simulink model "dual500MHzPFB"  (Simulink 6.2)
settings: Solver=ode45  StartTime=0.0  StopTime=10000  RelTol=1e-3
libraries: xbsIndex_r3 x2070, casper_library x180, xps_library x12, gtkWave x5, gavrt_library x1
(part 16 of 20)

== system dual500MHzPFB/cfgspec/FFT_Subsystem/fft_wideband_real1/fft_unscrambler/square_transposer/barrel_switcher ==
  sel : Inport  Port=1  LatchInput=off
  sync_in : Inport  Port=2  LatchInput=off
  In1 : Inport  Port=3  LatchInput=off
  In2 : Inport  Port=4  LatchInput=off
  Delay_sync : xbsIndex_r3/Delay  latency=1  reg_retiming=off  explicit_period=off  period=1  en=off  accept_only_valid=off  init_zero=on  dbl_ovrd=off  show_param=off
      settings: xl_area=[0, 0, 0, 0, 0, 0, 0]
  Mux11 : xbsIndex_r3/Mux  inputs=2  precision=Full  arith_type="Signed  (2's comp)"  n_bits=8  bin_pt=2  quantization=Truncate  overflow=Wrap  latency=1  explicit_period=off  period=1  en=off  dbl_ovrd=off  show_param=off  mux_type=off  use_rpm=off  gen_core=off
      settings: xl_area=[0, 0, 0, 0, 0, 0, 0]
  Mux21 : xbsIndex_r3/Mux  inputs=2  precision=Full  arith_type="Signed  (2's comp)"  n_bits=8  bin_pt=2  quantization=Truncate  overflow=Wrap  latency=1  explicit_period=off  period=1  en=off  dbl_ovrd=off  show_param=off  mux_type=off  use_rpm=off  gen_core=off
      settings: xl_area=[0, 0, 0, 0, 0, 0, 0]
  Slice1 : xbsIndex_r3/Slice  mode=Upper Bit Location + Width  nbits=1  bit1=-0  base1=MSB of Input  bit0=0  base0=LSB of Input  boolean_output=off  explicit_period=off  period=1  dbl_ovrd=off
  sync_out : Outport
  Out1 : Outport  Port=2
  Out2 : Outport  Port=3
  wires:
  Mux21/1 -> Out2/1
  In2/1 -> Mux11/3, Mux21/2
  Mux11/1 -> Out1/1
  In1/1 -> Mux21/3, Mux11/2
  Slice1/1 -> Mux21/1, Mux11/1
  sel/1 -> Slice1/1
  Delay_sync/1 -> sync_out/1
  sync_in/1 -> Delay_sync/1

== system dual500MHzPFB/cfgspec/PFB_Subsystem/pfb_fir_real/pol1_in1_last_tap/pfb_real_add_tree/adder_tree1 ==
  sync : Inport  Port=1  LatchInput=off
  din1 : Inport  Port=2  LatchInput=off
  din2 : Inport  Port=3  LatchInput=off
  addr1 : xbsIndex_r3/AddSub  mode=Addition  precision=Full  arith_type=Unsigned  n_bits=8  bin_pt=2  quantization=Truncate  overflow=Wrap  latency=2  explicit_period=off  period=1  use_carryin=off  use_carryout=off  en=off  dbl_ovrd=off  show_param=off  use_core=on  pipeline=on  use_rpm=on  gen_core=off
      settings: xl_area=[0, 0, 0, 0, 0, 0, 0]
  sync_delay : xbsIndex_r3/Delay  latency=2  reg_retiming=off  explicit_period=off  period=1  en=off  accept_only_valid=off  init_zero=on  dbl_ovrd=off  show_param=off
      settings: xl_area=[0, 0, 0, 0, 0, 0, 0]
  sync_out : Outport
  dout : Outport  Port=2
  wires:
  sync/1 -> sync_delay/1
  sync_delay/1 -> sync_out/1
  din1/1 -> addr1/1
  din2/1 -> addr1/2
  addr1/1 -> dout/1

== system dual500MHzPFB/cfgspec/PFB_Subsystem/pfb_fir_real/pol1_in2_last_tap/pfb_real_add_tree/adder_tree1 ==
  sync : Inport  Port=1  LatchInput=off
  din1 : Inport  Port=2  LatchInput=off
  din2 : Inport  Port=3  LatchInput=off
  addr1 : xbsIndex_r3/AddSub  mode=Addition  precision=Full  arith_type=Unsigned  n_bits=8  bin_pt=2  quantization=Truncate  overflow=Wrap  latency=2  explicit_period=off  period=1  use_carryin=off  use_carryout=off  en=off  dbl_ovrd=off  show_param=off  use_core=on  pipeline=on  use_rpm=on  gen_core=off
      settings: xl_area=[0, 0, 0, 0, 0, 0, 0]
  sync_delay : xbsIndex_r3/Delay  latency=2  reg_retiming=off  explicit_period=off  period=1  en=off  accept_only_valid=off  init_zero=on  dbl_ovrd=off  show_param=off
      settings: xl_area=[0, 0, 0, 0, 0, 0, 0]
  sync_out : Outport
  dout : Outport  Port=2
  wires:
  sync/1 -> sync_delay/1
  sync_delay/1 -> sync_out/1
  din1/1 -> addr1/1
  din2/1 -> addr1/2
  addr1/1 -> dout/1

== system dual500MHzPFB/cfgspec/PFB_Subsystem/pfb_fir_real/pol1_in3_last_tap/pfb_real_add_tree/adder_tree1 ==
  sync : Inport  Port=1  LatchInput=off
  din1 : Inport  Port=2  LatchInput=off
  din2 : Inport  Port=3  LatchInput=off
  addr1 : xbsIndex_r3/AddSub  mode=Addition  precision=Full  arith_type=Unsigned  n_bits=8  bin_pt=2  quantization=Truncate  overflow=Wrap  latency=2  explicit_period=off  period=1  use_carryin=off  use_carryout=off  en=off  dbl_ovrd=off  show_param=off  use_core=on  pipeline=on  use_rpm=on  gen_core=off
      settings: xl_area=[0, 0, 0, 0, 0, 0, 0]
  sync_delay : xbsIndex_r3/Delay  latency=2  reg_retiming=off  explicit_period=off  period=1  en=off  accept_only_valid=off  init_zero=on  dbl_ovrd=off  show_param=off
      settings: xl_area=[0, 0, 0, 0, 0, 0, 0]
  sync_out : Outport
  dout : Outport  Port=2
  wires:
  sync/1 -> sync_delay/1
  sync_delay/1 -> sync_out/1
  din1/1 -> addr1/1
  din2/1 -> addr1/2
  addr1/1 -> dout/1

== system dual500MHzPFB/cfgspec/PFB_Subsystem/pfb_fir_real/pol1_in4_last_tap/pfb_real_add_tree/adder_tree1 ==
  sync : Inport  Port=1  LatchInput=off
  din1 : Inport  Port=2  LatchInput=off
  din2 : Inport  Port=3  LatchInput=off
  addr1 : xbsIndex_r3/AddSub  mode=Addition  precision=Full  arith_type=Unsigned  n_bits=8  bin_pt=2  quantization=Truncate  overflow=Wrap  latency=2  explicit_period=off  period=1  use_carryin=off  use_carryout=off  en=off  dbl_ovrd=off  show_param=off  use_core=on  pipeline=on  use_rpm=on  gen_core=off
      settings: xl_area=[0, 0, 0, 0, 0, 0, 0]
  sync_delay : xbsIndex_r3/Delay  latency=2  reg_retiming=off  explicit_period=off  period=1  en=off  accept_only_valid=off  init_zero=on  dbl_ovrd=off  show_param=off
      settings: xl_area=[0, 0, 0, 0, 0, 0, 0]
  sync_out : Outport
  dout : Outport  Port=2
  wires:
  sync/1 -> sync_delay/1
  sync_delay/1 -> sync_out/1
  din1/1 -> addr1/1
  din2/1 -> addr1/2
  addr1/1 -> dout/1

== system dual500MHzPFB/cfgspec/PFB_Subsystem/pfb_fir_real1/pol1_in1_last_tap/pfb_real_add_tree/adder_tree1 ==
  sync : Inport  Port=1  LatchInput=off
  din1 : Inport  Port=2  LatchInput=off
  din2 : Inport  Port=3  LatchInput=off
  addr1 : xbsIndex_r3/AddSub  mode=Addition  precision=Full  arith_type=Unsigned  n_bits=8  bin_pt=2  quantization=Truncate  overflow=Wrap  latency=2  explicit_period=off  period=1  use_carryin=off  use_carryout=off  en=off  dbl_ovrd=off  show_param=off  use_core=on  pipeline=on  use_rpm=on  gen_core=off
      settings: xl_area=[0, 0, 0, 0, 0, 0, 0]
  sync_delay : xbsIndex_r3/Delay  latency=2  reg_retiming=off  explicit_period=off  period=1  en=off  accept_only_valid=off  init_zero=on  dbl_ovrd=off  show_param=off
      settings: xl_area=[0, 0, 0, 0, 0, 0, 0]
  sync_out : Outport
  dout : Outport  Port=2
  wires:
  sync/1 -> sync_delay/1
  sync_delay/1 -> sync_out/1
  din1/1 -> addr1/1
  din2/1 -> addr1/2
  addr1/1 -> dout/1

== system dual500MHzPFB/cfgspec/PFB_Subsystem/pfb_fir_real1/pol1_in2_last_tap/pfb_real_add_tree/adder_tree1 ==
  sync : Inport  Port=1  LatchInput=off
  din1 : Inport  Port=2  LatchInput=off
  din2 : Inport  Port=3  LatchInput=off
  addr1 : xbsIndex_r3/AddSub  mode=Addition  precision=Full  arith_type=Unsigned  n_bits=8  bin_pt=2  quantization=Truncate  overflow=Wrap  latency=2  explicit_period=off  period=1  use_carryin=off  use_carryout=off  en=off  dbl_ovrd=off  show_param=off  use_core=on  pipeline=on  use_rpm=on  gen_core=off
      settings: xl_area=[0, 0, 0, 0, 0, 0, 0]
  sync_delay : xbsIndex_r3/Delay  latency=2  reg_retiming=off  explicit_period=off  period=1  en=off  accept_only_valid=off  init_zero=on  dbl_ovrd=off  show_param=off
      settings: xl_area=[0, 0, 0, 0, 0, 0, 0]
  sync_out : Outport
  dout : Outport  Port=2
  wires:
  sync/1 -> sync_delay/1
  sync_delay/1 -> sync_out/1
  din1/1 -> addr1/1
  din2/1 -> addr1/2
  addr1/1 -> dout/1

== system dual500MHzPFB/cfgspec/PFB_Subsystem/pfb_fir_real1/pol1_in3_last_tap/pfb_real_add_tree/adder_tree1 ==
  sync : Inport  Port=1  LatchInput=off
  din1 : Inport  Port=2  LatchInput=off
  din2 : Inport  Port=3  LatchInput=off
  addr1 : xbsIndex_r3/AddSub  mode=Addition  precision=Full  arith_type=Unsigned  n_bits=8  bin_pt=2  quantization=Truncate  overflow=Wrap  latency=2  explicit_period=off  period=1  use_carryin=off  use_carryout=off  en=off  dbl_ovrd=off  show_param=off  use_core=on  pipeline=on  use_rpm=on  gen_core=off
      settings: xl_area=[0, 0, 0, 0, 0, 0, 0]
  sync_delay : xbsIndex_r3/Delay  latency=2  reg_retiming=off  explicit_period=off  period=1  en=off  accept_only_valid=off  init_zero=on  dbl_ovrd=off  show_param=off
      settings: xl_area=[0, 0, 0, 0, 0, 0, 0]
  sync_out : Outport
  dout : Outport  Port=2
  wires:
  sync/1 -> sync_delay/1
  sync_delay/1 -> sync_out/1
  din1/1 -> addr1/1
  din2/1 -> addr1/2
  addr1/1 -> dout/1

== system dual500MHzPFB/cfgspec/PFB_Subsystem/pfb_fir_real1/pol1_in4_last_tap/pfb_real_add_tree/adder_tree1 ==
  sync : Inport  Port=1  LatchInput=off
  din1 : Inport  Port=2  LatchInput=off
  din2 : Inport  Port=3  LatchInput=off
  addr1 : xbsIndex_r3/AddSub  mode=Addition  precision=Full  arith_type=Unsigned  n_bits=8  bin_pt=2  quantization=Truncate  overflow=Wrap  latency=2  explicit_period=off  period=1  use_carryin=off  use_carryout=off  en=off  dbl_ovrd=off  show_param=off  use_core=on  pipeline=on  use_rpm=on  gen_core=off
      settings: xl_area=[0, 0, 0, 0, 0, 0, 0]
  sync_delay : xbsIndex_r3/Delay  latency=2  reg_retiming=off  explicit_period=off  period=1  en=off  accept_only_valid=off  init_zero=on  dbl_ovrd=off  show_param=off
      settings: xl_area=[0, 0, 0, 0, 0, 0, 0]
  sync_out : Outport
  dout : Outport  Port=2
  wires:
  sync/1 -> sync_delay/1
  sync_delay/1 -> sync_out/1
  din1/1 -> addr1/1
  din2/1 -> addr1/2
  addr1/1 -> dout/1

== system dual500MHzPFB/cfgspec/FFT_Subsystem/fft_wideband_real/fft_biplex_real_4x0/biplex_core/fft_stage_1/butterfly ==
  a : Inport  Port=1  LatchInput=off
  b : Inport  Port=2  LatchInput=off
  sync : Inport  Port=3  LatchInput=off
  shift : Inport  Port=4  LatchInput=off
  AddSub : xbsIndex_r3/AddSub  mode=Addition  precision=Full  arith_type=Unsigned  n_bits=8  bin_pt=2  quantization=Truncate  overflow=Wrap  latency=add_latency  explicit_period=off  period=1  use_carryin=off  use_carryout=off  en=off  dbl_ovrd=off  show_param=on  use_core=on  pipeline=on  use_rpm=on  gen_core=on
      settings: xl_area=[0, 0, 0, 0, 0, 0, 0]
  AddSub1 : xbsIndex_r3/AddSub  mode=Addition  precision=Full  arith_type=Unsigned  n_bits=8  bin_pt=2  quantization=Truncate  overflow=Wrap  latency=add_latency  explicit_period=off  period=1  use_carryin=off  use_carryout=off  en=off  dbl_ovrd=off  show_param=on  use_core=on  pipeline=on  use_rpm=on  gen_core=on
      settings: xl_area=[0, 0, 0, 0, 0, 0, 0]
  AddSub2 : xbsIndex_r3/AddSub  mode=Subtraction  precision=Full  arith_type=Unsigned  n_bits=8  bin_pt=2  quantization=Truncate  overflow=Wrap  latency=add_latency  explicit_period=off  period=1  use_carryin=off  use_carryout=off  en=off  dbl_ovrd=off  show_param=on  use_core=on  pipeline=on  use_rpm=on  gen_core=on
      settings: xl_area=[0, 0, 0, 0, 0, 0, 0]
  AddSub3 : xbsIndex_r3/AddSub  mode=Subtraction  precision=Full  arith_type=Unsigned  n_bits=8  bin_pt=2  quantization=Truncate  overflow=Wrap  latency=add_latency  explicit_period=off  period=1  use_carryin=off  use_carryout=off  en=off  dbl_ovrd=off  show_param=on  use_core=on  pipeline=on  use_rpm=on  gen_core=on
      settings: xl_area=[0, 0, 0, 0, 0, 0, 0]
  Convert{,1..3} (4 alike) : xbsIndex_r3/Convert  arith_type="Signed  (2's comp)"  n_bits=BitWidth  bin_pt=BitWidth-1  quantization=Truncate  overflow=Wrap  latency=add_latency  explicit_period=off  period=1  dbl_ovrd=off  show_param=off  inserted_by_tool=off  pipeline=off
      settings: xl_area=[0, 0, 0, 0, 0, 0, 0]
  Delay : xbsIndex_r3/Delay  latency=2 * add_latency + 1  reg_retiming=off  explicit_period=off  period=1  en=off  accept_only_valid=off  init_zero=on  dbl_ovrd=off  show_param=off
      settings: xl_area=[0, 0, 0, 0, 0, 0, 0]
  Delay3 : xbsIndex_r3/Delay  latency=1  reg_retiming=off  explicit_period=off  period=1  en=off  accept_only_valid=off  init_zero=on  dbl_ovrd=off  show_param=off
      settings: xl_area=[0, 0, 0, 0, 0, 0, 0]
  Inverter : xbsIndex_r3/Inverter  latency=0  explicit_period=off  period=1  en=off  dbl_ovrd=off  show_param=off
      settings: xl_area=[0, 0, 0, 0, 0, 0, 0]
  Logical : xbsIndex_r3/Logical  logical_function=OR  inputs=4  precision=Full  arith_type=Unsigned  n_bits=8  bin_pt=2  align_bp=on  latency=1  explicit_period=off  period=1  en=off  dbl_ovrd=off  show_param=off
      settings: xl_area=[0, 0, 0, 0, 0, 0, 0]
  Logical{1,4,7,10} (4 alike) : xbsIndex_r3/Logical  logical_function=OR  inputs=2  precision=Full  arith_type=Unsigned  n_bits=8  bin_pt=2  align_bp=off  latency=1  explicit_period=off  period=1  en=off  dbl_ovrd=off  show_param=off
      settings: xl_area=[0, 0, 0, 0, 0, 0, 0]
  Logical{2,5,8,11} (4 alike) : xbsIndex_r3/Logical  logical_function=NOR  inputs=2  precision=Full  arith_type=Unsigned  n_bits=8  bin_pt=2  align_bp=off  latency=1  explicit_period=off  period=1  en=off  dbl_ovrd=off  show_param=off
      settings: xl_area=[0, 0, 0, 0, 0, 0, 0]
  Logical{3,6,9,12..13} (5 alike) : xbsIndex_r3/Logical  logical_function=AND  inputs=2  precision=Full  arith_type=Unsigned  n_bits=8  bin_pt=2  align_bp=off  latency=1  explicit_period=off  period=1  en=off  dbl_ovrd=off  show_param=off
      settings: xl_area=[0, 0, 0, 0, 0, 0, 0]
  Mux{,1..3} (4 alike) : xbsIndex_r3/Mux  inputs=2  precision=Full  arith_type="Signed  (2's comp)"  n_bits=8  bin_pt=2  quantization=Truncate  overflow=Wrap  latency=1  explicit_period=off  period=1  en=off  dbl_ovrd=off  show_param=off  mux_type=off  use_rpm=off  gen_core=off
      settings: xl_area=[0, 0, 0, 0, 0, 0, 0]
  Scale{,1..3} (4 alike) : xbsIndex_r3/Scale  scale_factor=-1  explicit_period=off  period=1  dbl_ovrd=off
  Slice{1,5,9,13} (4 alike) : xbsIndex_r3/Slice  mode=Upper Bit Location + Width  nbits=1  bit1=0  base1=MSB of Input  bit0=0  base0=LSB of Input  boolean_output=on  explicit_period=off  period=1  dbl_ovrd=off
  Slice{2,6,10,14} (4 alike) : xbsIndex_r3/Slice  mode=Upper Bit Location + Width  nbits=1  bit1=-1  base1=MSB of Input  bit0=0  base0=LSB of Input  boolean_output=on  explicit_period=off  period=1  dbl_ovrd=off
  c_to_ri : Subsystem
  c_to_ri1 : Subsystem
  ri_to_c : Subsystem
  ri_to_c1 : Subsystem
  a+bw : Outport
  a-bw : Outport  Port=2
  of : Outport  Port=3
  sync_out : Outport  Port=4
  wires:
  b/1 -> c_to_ri1/1(c)
  a/1 -> c_to_ri/1(c)
  sync/1 -> Delay/1
  c_to_ri1/2(im) -> AddSub3/2, AddSub1/2
  c_to_ri1/1(re) -> AddSub2/2, AddSub/2
  c_to_ri/2(im) -> AddSub3/1, AddSub1/1
  c_to_ri/1(re) -> AddSub2/1, AddSub/1
  ri_to_c/1(c) -> a+bw/1
  ri_to_c1/1(c) -> a-bw/1
  Delay/1 -> sync_out/1
  AddSub/1 -> Mux/2, Scale/1
  AddSub1/1 -> Mux1/2, Scale1/1
  shift/1 -> Delay3/1
  Mux/1 -> Convert/1, Slice2/1, Slice1/1
  Scale/1 -> Mux/3
  Convert/1 -> ri_to_c/1(re)
  Slice1/1 -> Logical3/1, Logical2/1
  Slice2/1 -> Logical3/2, Logical2/2
  Logical3/1 -> Logical1/1
  Logical2/1 -> Logical1/2
  Logical1/1 -> Logical/1
  Mux1/1 -> Convert1/1, Slice6/1, Slice5/1
  Scale1/1 -> Mux1/3
  Convert1/1 -> ri_to_c/2(im)
  Slice5/1 -> Logical6/1, Logical5/1
  Slice6/1 -> Logical6/2, Logical5/2
  Logical6/1 -> Logical4/1
  Logical5/1 -> Logical4/2
  Logical4/1 -> Logical/2
  Mux2/1 -> Convert2/1, Slice10/1, Slice9/1
  Scale2/1 -> Mux2/3
  Convert2/1 -> ri_to_c1/1(re)
  Slice9/1 -> Logical9/1, Logical8/1
  Slice10/1 -> Logical9/2, Logical8/2
  Logical9/1 -> Logical7/1
  Logical8/1 -> Logical7/2
  AddSub2/1 -> Mux2/2, Scale2/1
  Mux3/1 -> Convert3/1, Slice14/1, Slice13/1
  Scale3/1 -> Mux3/3
  Convert3/1 -> ri_to_c1/2(im)
  Slice13/1 -> Logical12/1, Logical11/1
  Slice14/1 -> Logical12/2, Logical11/2
  Logical12/1 -> Logical10/1
  Logical11/1 -> Logical10/2
  Logical10/1 -> Logical/4
  AddSub3/1 -> Mux3/2, Scale3/1
  Logical7/1 -> Logical/3
  Delay3/1 -> Mux/1, Mux1/1, Mux2/1, Mux3/1, Inverter/1
  Logical/1 -> Logical13/2
  Logical13/1 -> of/1
  Inverter/1 -> Logical13/1

== system dual500MHzPFB/cfgspec/FFT_Subsystem/fft_wideband_real/fft_biplex_real_4x0/biplex_core/fft_stage_1/delay_b ==
  In1 : Inport  Port=1  LatchInput=off
  delay_bram : casper_library/Delays/delay_bram  DelayLen=2^(FFTSize-FFTStage)  bram_latency=bram_latency
  Out1 : Outport
  wires:
  In1/1 -> delay_bram/1
  delay_bram/1 -> Out1/1

== system dual500MHzPFB/cfgspec/FFT_Subsystem/fft_wideband_real/fft_biplex_real_4x0/biplex_core/fft_stage_1/delay_f ==
  In1 : Inport  Port=1  LatchInput=off
  delay_bram : casper_library/Delays/delay_bram  DelayLen=2^(FFTSize-FFTStage)  bram_latency=bram_latency
  Out1 : Outport
  wires:
  In1/1 -> delay_bram/1
  delay_bram/1 -> Out1/1

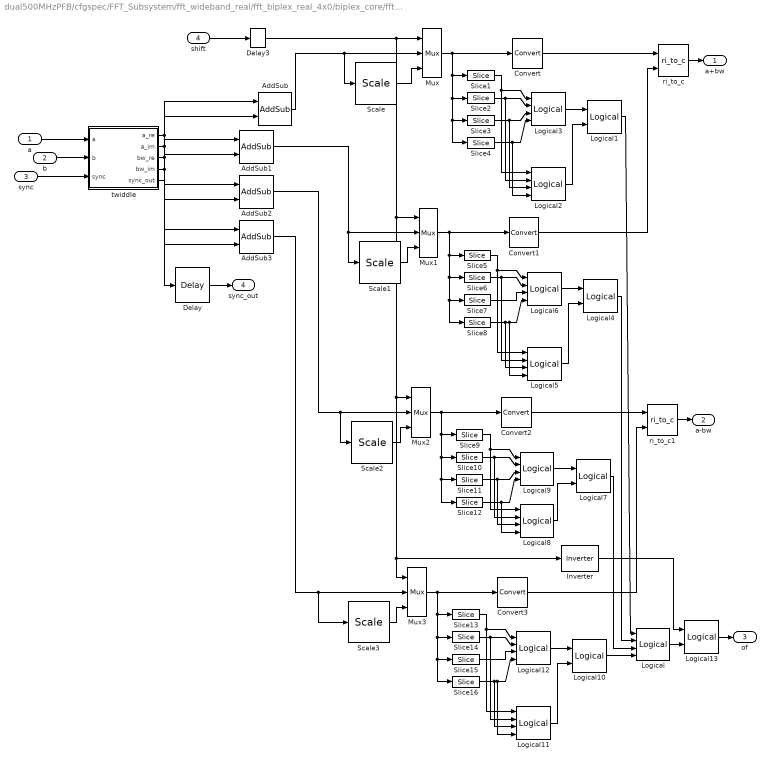
== system dual500MHzPFB/cfgspec/FFT_Subsystem/fft_wideband_real/fft_biplex_real_4x0/biplex_core/fft_stage_2/butterfly_direct ==
  a : Inport  Port=1  LatchInput=off
  b : Inport  Port=2  LatchInput=off
  sync : Inport  Port=3  LatchInput=off
  shift : Inport  Port=4  LatchInput=off
  AddSub : xbsIndex_r3/AddSub  mode=Addition  precision=Full  arith_type=Unsigned  n_bits=8  bin_pt=2  quantization=Truncate  overflow=Wrap  latency=add_latency  explicit_period=off  period=1  use_carryin=off  use_carryout=off  en=off  dbl_ovrd=off  show_param=on  use_core=on  pipeline=on  use_rpm=on  gen_core=on
      settings: xl_area=[0, 0, 0, 0, 0, 0, 0]
  AddSub1 : xbsIndex_r3/AddSub  mode=Addition  precision=Full  arith_type=Unsigned  n_bits=8  bin_pt=2  quantization=Truncate  overflow=Wrap  latency=add_latency  explicit_period=off  period=1  use_carryin=off  use_carryout=off  en=off  dbl_ovrd=off  show_param=on  use_core=on  pipeline=on  use_rpm=on  gen_core=on
      settings: xl_area=[0, 0, 0, 0, 0, 0, 0]
  AddSub2 : xbsIndex_r3/AddSub  mode=Subtraction  precision=Full  arith_type=Unsigned  n_bits=8  bin_pt=2  quantization=Truncate  overflow=Wrap  latency=add_latency  explicit_period=off  period=1  use_carryin=off  use_carryout=off  en=off  dbl_ovrd=off  show_param=on  use_core=on  pipeline=on  use_rpm=on  gen_core=on
      settings: xl_area=[0, 0, 0, 0, 0, 0, 0]
  AddSub3 : xbsIndex_r3/AddSub  mode=Subtraction  precision=Full  arith_type=Unsigned  n_bits=8  bin_pt=2  quantization=Truncate  overflow=Wrap  latency=add_latency  explicit_period=off  period=1  use_carryin=off  use_carryout=off  en=off  dbl_ovrd=off  show_param=on  use_core=on  pipeline=on  use_rpm=on  gen_core=on
      settings: xl_area=[0, 0, 0, 0, 0, 0, 0]
  Convert{,1..3} (4 alike) : xbsIndex_r3/Convert  arith_type="Signed  (2's comp)"  n_bits=BitWidth  bin_pt=BitWidth-1  quantization=Truncate  overflow=Wrap  latency=add_latency  explicit_period=off  period=1  dbl_ovrd=off  show_param=off  inserted_by_tool=off  pipeline=off
      settings: xl_area=[0, 0, 0, 0, 0, 0, 0]
  Delay : xbsIndex_r3/Delay  latency=2 * add_latency + 1  reg_retiming=off  explicit_period=off  period=1  en=off  accept_only_valid=off  init_zero=on  dbl_ovrd=off  show_param=off
      settings: xl_area=[0, 0, 0, 0, 0, 0, 0]
  Delay3 : xbsIndex_r3/Delay  latency=1  reg_retiming=off  explicit_period=off  period=1  en=off  accept_only_valid=off  init_zero=on  dbl_ovrd=off  show_param=off
      settings: xl_area=[0, 0, 0, 0, 0, 0, 0]
  Inverter : xbsIndex_r3/Inverter  latency=0  explicit_period=off  period=1  en=off  dbl_ovrd=off  show_param=off
      settings: xl_area=[0, 0, 0, 0, 0, 0, 0]
  Logical : xbsIndex_r3/Logical  logical_function=OR  inputs=4  precision=Full  arith_type=Unsigned  n_bits=8  bin_pt=2  align_bp=on  latency=1  explicit_period=off  period=1  en=off  dbl_ovrd=off  show_param=off
      settings: xl_area=[0, 0, 0, 0, 0, 0, 0]
  Logical{1,4,7,10} (4 alike) : xbsIndex_r3/Logical  logical_function=OR  inputs=2  precision=Full  arith_type=Unsigned  n_bits=8  bin_pt=2  align_bp=off  latency=1  explicit_period=off  period=1  en=off  dbl_ovrd=off  show_param=off
      settings: xl_area=[0, 0, 0, 0, 0, 0, 0]
  Logical{2,5,8,11} (4 alike) : xbsIndex_r3/Logical  logical_function=NOR  inputs=4  precision=Full  arith_type=Unsigned  n_bits=8  bin_pt=2  align_bp=off  latency=1  explicit_period=off  period=1  en=off  dbl_ovrd=off  show_param=off
      settings: xl_area=[0, 0, 0, 0, 0, 0, 0]
  Logical{3,6,9,12} (4 alike) : xbsIndex_r3/Logical  logical_function=AND  inputs=4  precision=Full  arith_type=Unsigned  n_bits=8  bin_pt=2  align_bp=off  latency=1  explicit_period=off  period=1  en=off  dbl_ovrd=off  show_param=off
      settings: xl_area=[0, 0, 0, 0, 0, 0, 0]
  Logical13 : xbsIndex_r3/Logical  logical_function=AND  inputs=2  precision=Full  arith_type=Unsigned  n_bits=8  bin_pt=2  align_bp=off  latency=1  explicit_period=off  period=1  en=off  dbl_ovrd=off  show_param=off
      settings: xl_area=[0, 0, 0, 0, 0, 0, 0]
  Mux{,1..3} (4 alike) : xbsIndex_r3/Mux  inputs=2  precision=Full  arith_type="Signed  (2's comp)"  n_bits=8  bin_pt=2  quantization=Truncate  overflow=Wrap  latency=1  explicit_period=off  period=1  en=off  dbl_ovrd=off  show_param=off  mux_type=off  use_rpm=off  gen_core=off
      settings: xl_area=[0, 0, 0, 0, 0, 0, 0]
  Scale{,1..3} (4 alike) : xbsIndex_r3/Scale  scale_factor=-1  explicit_period=off  period=1  dbl_ovrd=off
  Slice{1,5,9,13} (4 alike) : xbsIndex_r3/Slice  mode=Upper Bit Location + Width  nbits=1  bit1=0  base1=MSB of Input  bit0=0  base0=LSB of Input  boolean_output=on  explicit_period=off  period=1  dbl_ovrd=off
  Slice{2,6,10,14} (4 alike) : xbsIndex_r3/Slice  mode=Upper Bit Location + Width  nbits=1  bit1=-1  base1=MSB of Input  bit0=0  base0=LSB of Input  boolean_output=on  explicit_period=off  period=1  dbl_ovrd=off
  Slice{3,7,11,15} (4 alike) : xbsIndex_r3/Slice  mode=Upper Bit Location + Width  nbits=1  bit1=-2  base1=MSB of Input  bit0=0  base0=LSB of Input  boolean_output=on  explicit_period=off  period=1  dbl_ovrd=off
  Slice{4,8,12,16} (4 alike) : xbsIndex_r3/Slice  mode=Upper Bit Location + Width  nbits=1  bit1=-3  base1=MSB of Input  bit0=0  base0=LSB of Input  boolean_output=on  explicit_period=off  period=1  dbl_ovrd=off
  ri_to_c : casper_library/Misc/ri_to_c
  ri_to_c1 : casper_library/Misc/ri_to_c
  twiddle : Subsystem  BlockChoice=twiddle_stage_2
      link override twiddle_general_3mult: Coeffs="[1+0i           6.1232e-017-1i          ]"  StepPeriod=5  BitWidth=18  add_latency=3  mult_latency=3  bram_latency=2
      link override twiddle_general_3mult/coeff_gen: BlockChoice=br_coeff_gen
      link override twiddle_general_3mult/coeff_gen/br_coeff_gen: Coeffs=[1 2 3 4 5 6 7]  StepPeriod=4  BitWidth=10  bram_latency=6
      link override twiddle_general_3mult/coeff_gen/br_coeff_gen/ROM: distributed_mem=off
      link override twiddle_general_3mult/coeff_gen/br_coeff_gen/ROM1: distributed_mem=off
      link override twiddle_stage_2: FFTSize=8  BitWidth=18  add_latency=3  mult_latency=3  bram_latency=2
      settings: AttributesFormatString=%<BlockChoice>  TemplateBlock=casper_library/FFTs/Twiddle/twiddle  MemberBlocks=twiddle_coeff_0,twiddle_coeff_1,twiddle_general_3mult,twiddle_general_4mult,twiddle_stage_2
  a+bw : Outport
  a-bw : Outport  Port=2
  of : Outport  Port=3
  sync_out : Outport  Port=4
  wires:
  Inverter/1 -> Logical13/1
  Logical13/1 -> of/1
  Logical/1 -> Logical13/2
  Delay3/1 -> Inverter/1, Mux3/1, Mux2/1, Mux1/1, Mux/1
  Logical7/1 -> Logical/3
  AddSub3/1 -> Scale3/1, Mux3/2
  Logical10/1 -> Logical/4
  Logical11/1 -> Logical10/2
  Logical12/1 -> Logical10/1
  Slice16/1 -> Logical11/3, Logical11/4, Logical12/4
  Slice15/1 -> Logical12/3
  Slice14/1 -> Logical11/2, Logical12/2
  Slice13/1 -> Logical11/1, Logical12/1
  Convert3/1 -> ri_to_c1/2
  Scale3/1 -> Mux3/3
  Mux3/1 -> Slice16/1, Slice15/1, Slice14/1, Slice13/1, Convert3/1
  AddSub2/1 -> Scale2/1, Mux2/2
  Logical8/1 -> Logical7/2
  Logical9/1 -> Logical7/1
  Slice12/1 -> Logical8/4, Logical9/4
  Slice11/1 -> Logical8/3, Logical9/3
  Slice10/1 -> Logical8/2, Logical9/2
  Slice9/1 -> Logical8/1, Logical9/1
  Convert2/1 -> ri_to_c1/1
  Scale2/1 -> Mux2/3
  Mux2/1 -> Slice12/1, Slice11/1, Slice10/1, Slice9/1, Convert2/1
  Logical4/1 -> Logical/2
  Logical5/1 -> Logical4/2
  Logical6/1 -> Logical4/1
  Slice8/1 -> Logical5/3, Logical5/4, Logical6/4
  Slice7/1 -> Logical6/3
  Slice6/1 -> Logical5/2, Logical6/2
  Slice5/1 -> Logical5/1, Logical6/1
  Convert1/1 -> ri_to_c/2
  Scale1/1 -> Mux1/3
  Mux1/1 -> Slice8/1, Slice7/1, Slice6/1, Slice5/1, Convert1/1
  Logical1/1 -> Logical/1
  Logical2/1 -> Logical1/2
  Logical3/1 -> Logical1/1
  Slice4/1 -> Logical2/4, Logical3/4
  Slice3/1 -> Logical2/3, Logical3/3
  Slice2/1 -> Logical2/2, Logical3/2
  Slice1/1 -> Logical2/1, Logical3/1
  Convert/1 -> ri_to_c/1
  Scale/1 -> Mux/3
  Mux/1 -> Slice4/1, Slice3/1, Slice2/1, Slice1/1, Convert/1
  shift/1 -> Delay3/1
  AddSub1/1 -> Scale1/1, Mux1/2
  AddSub/1 -> Scale/1, Mux/2
  Delay/1 -> sync_out/1
  ri_to_c1/1 -> a-bw/1
  ri_to_c/1 -> a+bw/1
  a/1 -> twiddle/1(a)
  b/1 -> twiddle/2(b)
  sync/1 -> twiddle/3(sync)
  twiddle/1(a_re) -> AddSub/1, AddSub2/1
  twiddle/2(a_im) -> AddSub1/1, AddSub3/1
  twiddle/3(bw_re) -> AddSub/2, AddSub2/2
  twiddle/4(bw_im) -> AddSub1/2, AddSub3/2
  twiddle/5(sync_out) -> Delay/1

== system dual500MHzPFB/cfgspec/FFT_Subsystem/fft_wideband_real/fft_biplex_real_4x0/biplex_core/fft_stage_2/delay_b ==
  In1 : Inport  Port=1  LatchInput=off
  delay_bram : casper_library/Delays/delay_bram  DelayLen=2^(FFTSize-FFTStage)  bram_latency=bram_latency
  Out1 : Outport
  wires:
  In1/1 -> delay_bram/1
  delay_bram/1 -> Out1/1

== system dual500MHzPFB/cfgspec/FFT_Subsystem/fft_wideband_real/fft_biplex_real_4x0/biplex_core/fft_stage_2/delay_f ==
  In1 : Inport  Port=1  LatchInput=off
  delay_bram : casper_library/Delays/delay_bram  DelayLen=2^(FFTSize-FFTStage)  bram_latency=bram_latency
  Out1 : Outport
  wires:
  In1/1 -> delay_bram/1
  delay_bram/1 -> Out1/1

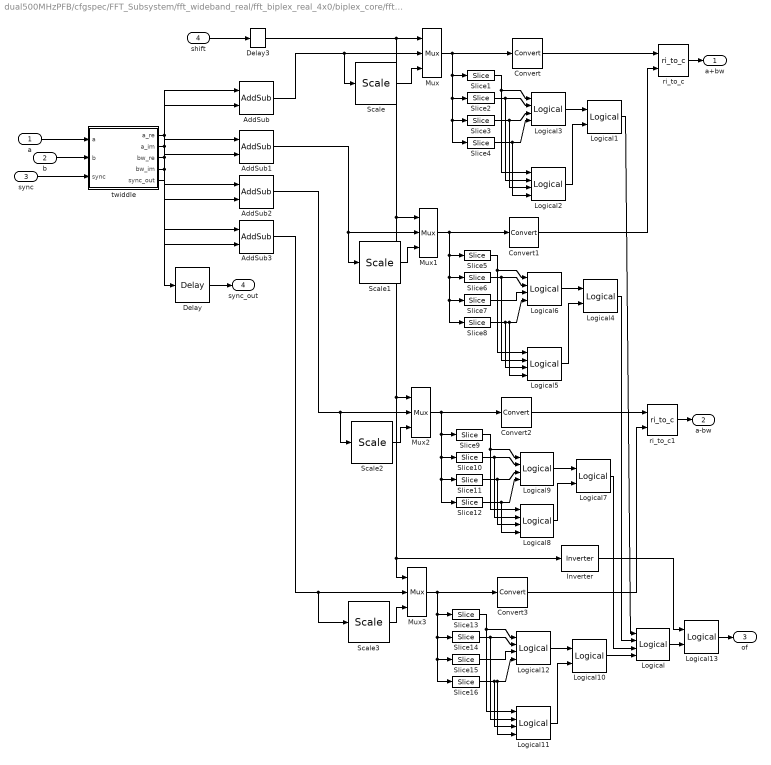
== system dual500MHzPFB/cfgspec/FFT_Subsystem/fft_wideband_real/fft_biplex_real_4x0/biplex_core/fft_stage_3/butterfly_direct ==
  a : Inport  Port=1  LatchInput=off
  b : Inport  Port=2  LatchInput=off
  sync : Inport  Port=3  LatchInput=off
  shift : Inport  Port=4  LatchInput=off
  AddSub : xbsIndex_r3/AddSub  mode=Addition  precision=Full  arith_type=Unsigned  n_bits=8  bin_pt=2  quantization=Truncate  overflow=Wrap  latency=add_latency  explicit_period=off  period=1  use_carryin=off  use_carryout=off  en=off  dbl_ovrd=off  show_param=on  use_core=on  pipeline=on  use_rpm=on  gen_core=on
      settings: xl_area=[0, 0, 0, 0, 0, 0, 0]
  AddSub1 : xbsIndex_r3/AddSub  mode=Addition  precision=Full  arith_type=Unsigned  n_bits=8  bin_pt=2  quantization=Truncate  overflow=Wrap  latency=add_latency  explicit_period=off  period=1  use_carryin=off  use_carryout=off  en=off  dbl_ovrd=off  show_param=on  use_core=on  pipeline=on  use_rpm=on  gen_core=on
      settings: xl_area=[0, 0, 0, 0, 0, 0, 0]
  AddSub2 : xbsIndex_r3/AddSub  mode=Subtraction  precision=Full  arith_type=Unsigned  n_bits=8  bin_pt=2  quantization=Truncate  overflow=Wrap  latency=add_latency  explicit_period=off  period=1  use_carryin=off  use_carryout=off  en=off  dbl_ovrd=off  show_param=on  use_core=on  pipeline=on  use_rpm=on  gen_core=on
      settings: xl_area=[0, 0, 0, 0, 0, 0, 0]
  AddSub3 : xbsIndex_r3/AddSub  mode=Subtraction  precision=Full  arith_type=Unsigned  n_bits=8  bin_pt=2  quantization=Truncate  overflow=Wrap  latency=add_latency  explicit_period=off  period=1  use_carryin=off  use_carryout=off  en=off  dbl_ovrd=off  show_param=on  use_core=on  pipeline=on  use_rpm=on  gen_core=on
      settings: xl_area=[0, 0, 0, 0, 0, 0, 0]
  Convert{,1..3} (4 alike) : xbsIndex_r3/Convert  arith_type="Signed  (2's comp)"  n_bits=BitWidth  bin_pt=BitWidth-1  quantization=Truncate  overflow=Wrap  latency=add_latency  explicit_period=off  period=1  dbl_ovrd=off  show_param=off  inserted_by_tool=off  pipeline=off
      settings: xl_area=[0, 0, 0, 0, 0, 0, 0]
  Delay : xbsIndex_r3/Delay  latency=2 * add_latency + 1  reg_retiming=off  explicit_period=off  period=1  en=off  accept_only_valid=off  init_zero=on  dbl_ovrd=off  show_param=off
      settings: xl_area=[0, 0, 0, 0, 0, 0, 0]
  Delay3 : xbsIndex_r3/Delay  latency=1  reg_retiming=off  explicit_period=off  period=1  en=off  accept_only_valid=off  init_zero=on  dbl_ovrd=off  show_param=off
      settings: xl_area=[0, 0, 0, 0, 0, 0, 0]
  Inverter : xbsIndex_r3/Inverter  latency=0  explicit_period=off  period=1  en=off  dbl_ovrd=off  show_param=off
      settings: xl_area=[0, 0, 0, 0, 0, 0, 0]
  Logical : xbsIndex_r3/Logical  logical_function=OR  inputs=4  precision=Full  arith_type=Unsigned  n_bits=8  bin_pt=2  align_bp=on  latency=1  explicit_period=off  period=1  en=off  dbl_ovrd=off  show_param=off
      settings: xl_area=[0, 0, 0, 0, 0, 0, 0]
  Logical{1,4,7,10} (4 alike) : xbsIndex_r3/Logical  logical_function=OR  inputs=2  precision=Full  arith_type=Unsigned  n_bits=8  bin_pt=2  align_bp=off  latency=1  explicit_period=off  period=1  en=off  dbl_ovrd=off  show_param=off
      settings: xl_area=[0, 0, 0, 0, 0, 0, 0]
  Logical{2,5,8,11} (4 alike) : xbsIndex_r3/Logical  logical_function=NOR  inputs=4  precision=Full  arith_type=Unsigned  n_bits=8  bin_pt=2  align_bp=off  latency=1  explicit_period=off  period=1  en=off  dbl_ovrd=off  show_param=off
      settings: xl_area=[0, 0, 0, 0, 0, 0, 0]
  Logical{3,6,9,12} (4 alike) : xbsIndex_r3/Logical  logical_function=AND  inputs=4  precision=Full  arith_type=Unsigned  n_bits=8  bin_pt=2  align_bp=off  latency=1  explicit_period=off  period=1  en=off  dbl_ovrd=off  show_param=off
      settings: xl_area=[0, 0, 0, 0, 0, 0, 0]
  Logical13 : xbsIndex_r3/Logical  logical_function=AND  inputs=2  precision=Full  arith_type=Unsigned  n_bits=8  bin_pt=2  align_bp=off  latency=1  explicit_period=off  period=1  en=off  dbl_ovrd=off  show_param=off
      settings: xl_area=[0, 0, 0, 0, 0, 0, 0]
  Mux{,1..3} (4 alike) : xbsIndex_r3/Mux  inputs=2  precision=Full  arith_type="Signed  (2's comp)"  n_bits=8  bin_pt=2  quantization=Truncate  overflow=Wrap  latency=1  explicit_period=off  period=1  en=off  dbl_ovrd=off  show_param=off  mux_type=off  use_rpm=off  gen_core=off
      settings: xl_area=[0, 0, 0, 0, 0, 0, 0]
  Scale{,1..3} (4 alike) : xbsIndex_r3/Scale  scale_factor=-1  explicit_period=off  period=1  dbl_ovrd=off
  Slice{1,5,9,13} (4 alike) : xbsIndex_r3/Slice  mode=Upper Bit Location + Width  nbits=1  bit1=0  base1=MSB of Input  bit0=0  base0=LSB of Input  boolean_output=on  explicit_period=off  period=1  dbl_ovrd=off
  Slice{2,6,10,14} (4 alike) : xbsIndex_r3/Slice  mode=Upper Bit Location + Width  nbits=1  bit1=-1  base1=MSB of Input  bit0=0  base0=LSB of Input  boolean_output=on  explicit_period=off  period=1  dbl_ovrd=off
  Slice{3,7,11,15} (4 alike) : xbsIndex_r3/Slice  mode=Upper Bit Location + Width  nbits=1  bit1=-2  base1=MSB of Input  bit0=0  base0=LSB of Input  boolean_output=on  explicit_period=off  period=1  dbl_ovrd=off
  Slice{4,8,12,16} (4 alike) : xbsIndex_r3/Slice  mode=Upper Bit Location + Width  nbits=1  bit1=-3  base1=MSB of Input  bit0=0  base0=LSB of Input  boolean_output=on  explicit_period=off  period=1  dbl_ovrd=off
  ri_to_c : casper_library/Misc/ri_to_c
  ri_to_c1 : casper_library/Misc/ri_to_c
  twiddle : Subsystem  BlockChoice=twiddle_general_3mult
      link override twiddle_general_3mult: Coeffs="[1+0i           6.1232e-017-1i               0.70711-0.70711i        -0.70711-0.70711i    ]"  StepPeriod=5  BitWidth=18  add_latency=3  mult_latency=3  bram_latency=2
      link override twiddle_general_3mult/coeff_gen: BlockChoice=br_coeff_gen
      link override twiddle_general_3mult/coeff_gen/br_coeff_gen: Coeffs=[1 2 3 4 5 6 7]  StepPeriod=4  BitWidth=10  bram_latency=6
      link override twiddle_general_3mult/coeff_gen/br_coeff_gen/ROM: distributed_mem=off
      link override twiddle_general_3mult/coeff_gen/br_coeff_gen/ROM1: distributed_mem=off
      link override twiddle_general_3mult/coeff_gen/static_coeff_gen/Constant: equ=P=C
      link override twiddle_general_3mult/coeff_gen/static_coeff_gen/Constant1: equ=P=C
      settings: AttributesFormatString=%<BlockChoice>  TemplateBlock=casper_library/FFTs/Twiddle/twiddle  MemberBlocks=twiddle_coeff_0,twiddle_coeff_1,twiddle_general_3mult,twiddle_general_4mult,twiddle_stage_2
  a+bw : Outport
  a-bw : Outport  Port=2
  of : Outport  Port=3
  sync_out : Outport  Port=4
  wires:
  Inverter/1 -> Logical13/1
  Logical13/1 -> of/1
  Logical/1 -> Logical13/2
  Delay3/1 -> Inverter/1, Mux3/1, Mux2/1, Mux1/1, Mux/1
  Logical7/1 -> Logical/3
  AddSub3/1 -> Scale3/1, Mux3/2
  Logical10/1 -> Logical/4
  Logical11/1 -> Logical10/2
  Logical12/1 -> Logical10/1
  Slice16/1 -> Logical11/3, Logical11/4, Logical12/4
  Slice15/1 -> Logical12/3
  Slice14/1 -> Logical11/2, Logical12/2
  Slice13/1 -> Logical11/1, Logical12/1
  Convert3/1 -> ri_to_c1/2
  Scale3/1 -> Mux3/3
  Mux3/1 -> Slice16/1, Slice15/1, Slice14/1, Slice13/1, Convert3/1
  AddSub2/1 -> Scale2/1, Mux2/2
  Logical8/1 -> Logical7/2
  Logical9/1 -> Logical7/1
  Slice12/1 -> Logical8/4, Logical9/4
  Slice11/1 -> Logical8/3, Logical9/3
  Slice10/1 -> Logical8/2, Logical9/2
  Slice9/1 -> Logical8/1, Logical9/1
  Convert2/1 -> ri_to_c1/1
  Scale2/1 -> Mux2/3
  Mux2/1 -> Slice12/1, Slice11/1, Slice10/1, Slice9/1, Convert2/1
  Logical4/1 -> Logical/2
  Logical5/1 -> Logical4/2
  Logical6/1 -> Logical4/1
  Slice8/1 -> Logical5/3, Logical5/4, Logical6/4
  Slice7/1 -> Logical6/3
  Slice6/1 -> Logical5/2, Logical6/2
  Slice5/1 -> Logical5/1, Logical6/1
  Convert1/1 -> ri_to_c/2
  Scale1/1 -> Mux1/3
  Mux1/1 -> Slice8/1, Slice7/1, Slice6/1, Slice5/1, Convert1/1
  Logical1/1 -> Logical/1
  Logical2/1 -> Logical1/2
  Logical3/1 -> Logical1/1
  Slice4/1 -> Logical2/4, Logical3/4
  Slice3/1 -> Logical2/3, Logical3/3
  Slice2/1 -> Logical2/2, Logical3/2
  Slice1/1 -> Logical2/1, Logical3/1
  Convert/1 -> ri_to_c/1
  Scale/1 -> Mux/3
  Mux/1 -> Slice4/1, Slice3/1, Slice2/1, Slice1/1, Convert/1
  shift/1 -> Delay3/1
  AddSub1/1 -> Scale1/1, Mux1/2
  AddSub/1 -> Scale/1, Mux/2
  Delay/1 -> sync_out/1
  ri_to_c1/1 -> a-bw/1
  ri_to_c/1 -> a+bw/1
  a/1 -> twiddle/1(a)
  b/1 -> twiddle/2(b)
  sync/1 -> twiddle/3(sync)
  twiddle/1(a_re) -> AddSub/1, AddSub2/1
  twiddle/2(a_im) -> AddSub1/1, AddSub3/1
  twiddle/3(bw_re) -> AddSub/2, AddSub2/2
  twiddle/4(bw_im) -> AddSub1/2, AddSub3/2
  twiddle/5(sync_out) -> Delay/1

== system dual500MHzPFB/cfgspec/FFT_Subsystem/fft_wideband_real/fft_biplex_real_4x0/biplex_core/fft_stage_3/delay_b ==
  In1 : Inport  Port=1  LatchInput=off
  delay_slr : casper_library/Delays/delay_slr  DelayLen=2^(FFTSize-FFTStage)
  Out1 : Outport
  wires:
  In1/1 -> delay_slr/1
  delay_slr/1 -> Out1/1

== system dual500MHzPFB/cfgspec/FFT_Subsystem/fft_wideband_real/fft_biplex_real_4x0/biplex_core/fft_stage_3/delay_f ==
  In1 : Inport  Port=1  LatchInput=off
  delay_slr : casper_library/Delays/delay_slr  DelayLen=2^(FFTSize-FFTStage)
  Out1 : Outport
  wires:
  In1/1 -> delay_slr/1
  delay_slr/1 -> Out1/1

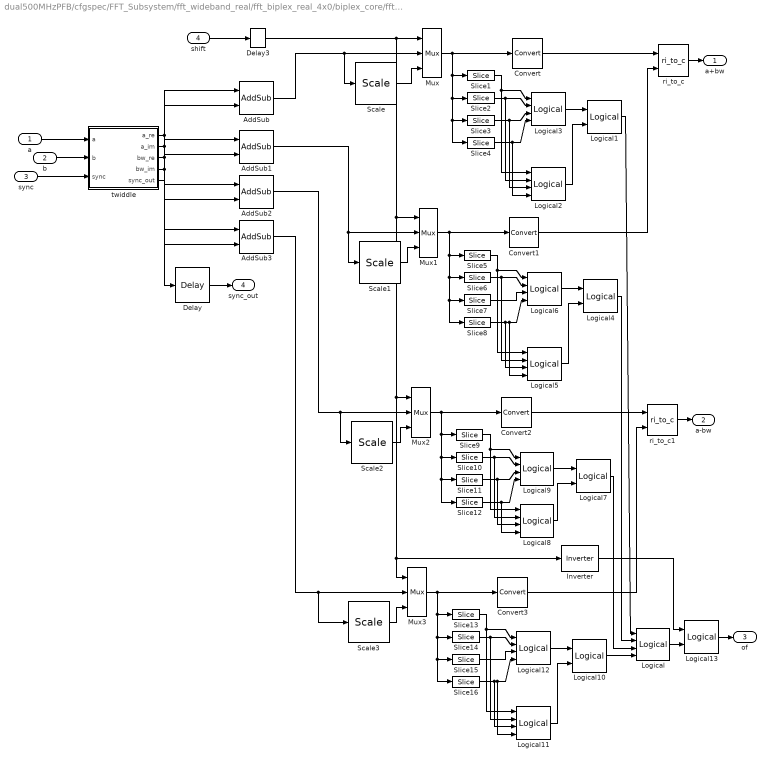
== system dual500MHzPFB/cfgspec/FFT_Subsystem/fft_wideband_real/fft_biplex_real_4x0/biplex_core/fft_stage_4/butterfly_direct ==
  a : Inport  Port=1  LatchInput=off
  b : Inport  Port=2  LatchInput=off
  sync : Inport  Port=3  LatchInput=off
  shift : Inport  Port=4  LatchInput=off
  AddSub : xbsIndex_r3/AddSub  mode=Addition  precision=Full  arith_type=Unsigned  n_bits=8  bin_pt=2  quantization=Truncate  overflow=Wrap  latency=add_latency  explicit_period=off  period=1  use_carryin=off  use_carryout=off  en=off  dbl_ovrd=off  show_param=on  use_core=on  pipeline=on  use_rpm=on  gen_core=on
      settings: xl_area=[0, 0, 0, 0, 0, 0, 0]
  AddSub1 : xbsIndex_r3/AddSub  mode=Addition  precision=Full  arith_type=Unsigned  n_bits=8  bin_pt=2  quantization=Truncate  overflow=Wrap  latency=add_latency  explicit_period=off  period=1  use_carryin=off  use_carryout=off  en=off  dbl_ovrd=off  show_param=on  use_core=on  pipeline=on  use_rpm=on  gen_core=on
      settings: xl_area=[0, 0, 0, 0, 0, 0, 0]
  AddSub2 : xbsIndex_r3/AddSub  mode=Subtraction  precision=Full  arith_type=Unsigned  n_bits=8  bin_pt=2  quantization=Truncate  overflow=Wrap  latency=add_latency  explicit_period=off  period=1  use_carryin=off  use_carryout=off  en=off  dbl_ovrd=off  show_param=on  use_core=on  pipeline=on  use_rpm=on  gen_core=on
      settings: xl_area=[0, 0, 0, 0, 0, 0, 0]
  AddSub3 : xbsIndex_r3/AddSub  mode=Subtraction  precision=Full  arith_type=Unsigned  n_bits=8  bin_pt=2  quantization=Truncate  overflow=Wrap  latency=add_latency  explicit_period=off  period=1  use_carryin=off  use_carryout=off  en=off  dbl_ovrd=off  show_param=on  use_core=on  pipeline=on  use_rpm=on  gen_core=on
      settings: xl_area=[0, 0, 0, 0, 0, 0, 0]
  Convert{,1..3} (4 alike) : xbsIndex_r3/Convert  arith_type="Signed  (2's comp)"  n_bits=BitWidth  bin_pt=BitWidth-1  quantization=Truncate  overflow=Wrap  latency=add_latency  explicit_period=off  period=1  dbl_ovrd=off  show_param=off  inserted_by_tool=off  pipeline=off
      settings: xl_area=[0, 0, 0, 0, 0, 0, 0]
  Delay : xbsIndex_r3/Delay  latency=2 * add_latency + 1  reg_retiming=off  explicit_period=off  period=1  en=off  accept_only_valid=off  init_zero=on  dbl_ovrd=off  show_param=off
      settings: xl_area=[0, 0, 0, 0, 0, 0, 0]
  Delay3 : xbsIndex_r3/Delay  latency=1  reg_retiming=off  explicit_period=off  period=1  en=off  accept_only_valid=off  init_zero=on  dbl_ovrd=off  show_param=off
      settings: xl_area=[0, 0, 0, 0, 0, 0, 0]
  Inverter : xbsIndex_r3/Inverter  latency=0  explicit_period=off  period=1  en=off  dbl_ovrd=off  show_param=off
      settings: xl_area=[0, 0, 0, 0, 0, 0, 0]
  Logical : xbsIndex_r3/Logical  logical_function=OR  inputs=4  precision=Full  arith_type=Unsigned  n_bits=8  bin_pt=2  align_bp=on  latency=1  explicit_period=off  period=1  en=off  dbl_ovrd=off  show_param=off
      settings: xl_area=[0, 0, 0, 0, 0, 0, 0]
  Logical{1,4,7,10} (4 alike) : xbsIndex_r3/Logical  logical_function=OR  inputs=2  precision=Full  arith_type=Unsigned  n_bits=8  bin_pt=2  align_bp=off  latency=1  explicit_period=off  period=1  en=off  dbl_ovrd=off  show_param=off
      settings: xl_area=[0, 0, 0, 0, 0, 0, 0]
  Logical{2,5,8,11} (4 alike) : xbsIndex_r3/Logical  logical_function=NOR  inputs=4  precision=Full  arith_type=Unsigned  n_bits=8  bin_pt=2  align_bp=off  latency=1  explicit_period=off  period=1  en=off  dbl_ovrd=off  show_param=off
      settings: xl_area=[0, 0, 0, 0, 0, 0, 0]
  Logical{3,6,9,12} (4 alike) : xbsIndex_r3/Logical  logical_function=AND  inputs=4  precision=Full  arith_type=Unsigned  n_bits=8  bin_pt=2  align_bp=off  latency=1  explicit_period=off  period=1  en=off  dbl_ovrd=off  show_param=off
      settings: xl_area=[0, 0, 0, 0, 0, 0, 0]
  Logical13 : xbsIndex_r3/Logical  logical_function=AND  inputs=2  precision=Full  arith_type=Unsigned  n_bits=8  bin_pt=2  align_bp=off  latency=1  explicit_period=off  period=1  en=off  dbl_ovrd=off  show_param=off
      settings: xl_area=[0, 0, 0, 0, 0, 0, 0]
  Mux{,1..3} (4 alike) : xbsIndex_r3/Mux  inputs=2  precision=Full  arith_type="Signed  (2's comp)"  n_bits=8  bin_pt=2  quantization=Truncate  overflow=Wrap  latency=1  explicit_period=off  period=1  en=off  dbl_ovrd=off  show_param=off  mux_type=off  use_rpm=off  gen_core=off
      settings: xl_area=[0, 0, 0, 0, 0, 0, 0]
  Scale{,1..3} (4 alike) : xbsIndex_r3/Scale  scale_factor=-1  explicit_period=off  period=1  dbl_ovrd=off
  Slice{1,5,9,13} (4 alike) : xbsIndex_r3/Slice  mode=Upper Bit Location + Width  nbits=1  bit1=0  base1=MSB of Input  bit0=0  base0=LSB of Input  boolean_output=on  explicit_period=off  period=1  dbl_ovrd=off
  Slice{2,6,10,14} (4 alike) : xbsIndex_r3/Slice  mode=Upper Bit Location + Width  nbits=1  bit1=-1  base1=MSB of Input  bit0=0  base0=LSB of Input  boolean_output=on  explicit_period=off  period=1  dbl_ovrd=off
  Slice{3,7,11,15} (4 alike) : xbsIndex_r3/Slice  mode=Upper Bit Location + Width  nbits=1  bit1=-2  base1=MSB of Input  bit0=0  base0=LSB of Input  boolean_output=on  explicit_period=off  period=1  dbl_ovrd=off
  Slice{4,8,12,16} (4 alike) : xbsIndex_r3/Slice  mode=Upper Bit Location + Width  nbits=1  bit1=-3  base1=MSB of Input  bit0=0  base0=LSB of Input  boolean_output=on  explicit_period=off  period=1  dbl_ovrd=off
  ri_to_c : casper_library/Misc/ri_to_c
  ri_to_c1 : casper_library/Misc/ri_to_c
  twiddle : Subsystem  BlockChoice=twiddle_general_3mult
      link override twiddle_general_3mult: Coeffs="[1+0i           6.1232e-017-1i               0.70711-0.70711i        -0.70711-0.70711i         0.92388-0.38268i        -0.38268-0.92388i         0.38268-0.92388i        -0.92388-0.38268i    ]"  StepPeriod=4  BitWidth=18  add_latency=3  mult_latency=3  bram_latency=2
      link override twiddle_general_3mult/coeff_gen: BlockChoice=br_coeff_gen
      link override twiddle_general_3mult/coeff_gen/br_coeff_gen: Coeffs=[1 2 3 4 5 6 7]  StepPeriod=4  BitWidth=10  bram_latency=6
      link override twiddle_general_3mult/coeff_gen/br_coeff_gen/ROM: distributed_mem=off
      link override twiddle_general_3mult/coeff_gen/br_coeff_gen/ROM1: distributed_mem=off
      link override twiddle_general_3mult/coeff_gen/static_coeff_gen/Constant: equ=P=C
      link override twiddle_general_3mult/coeff_gen/static_coeff_gen/Constant1: equ=P=C
      settings: AttributesFormatString=%<BlockChoice>  TemplateBlock=casper_library/FFTs/Twiddle/twiddle  MemberBlocks=twiddle_coeff_0,twiddle_coeff_1,twiddle_general_3mult,twiddle_general_4mult,twiddle_stage_2
  a+bw : Outport
  a-bw : Outport  Port=2
  of : Outport  Port=3
  sync_out : Outport  Port=4
  wires:
  Inverter/1 -> Logical13/1
  Logical13/1 -> of/1
  Logical/1 -> Logical13/2
  Delay3/1 -> Inverter/1, Mux3/1, Mux2/1, Mux1/1, Mux/1
  Logical7/1 -> Logical/3
  AddSub3/1 -> Scale3/1, Mux3/2
  Logical10/1 -> Logical/4
  Logical11/1 -> Logical10/2
  Logical12/1 -> Logical10/1
  Slice16/1 -> Logical11/3, Logical11/4, Logical12/4
  Slice15/1 -> Logical12/3
  Slice14/1 -> Logical11/2, Logical12/2
  Slice13/1 -> Logical11/1, Logical12/1
  Convert3/1 -> ri_to_c1/2
  Scale3/1 -> Mux3/3
  Mux3/1 -> Slice16/1, Slice15/1, Slice14/1, Slice13/1, Convert3/1
  AddSub2/1 -> Scale2/1, Mux2/2
  Logical8/1 -> Logical7/2
  Logical9/1 -> Logical7/1
  Slice12/1 -> Logical8/4, Logical9/4
  Slice11/1 -> Logical8/3, Logical9/3
  Slice10/1 -> Logical8/2, Logical9/2
  Slice9/1 -> Logical8/1, Logical9/1
  Convert2/1 -> ri_to_c1/1
  Scale2/1 -> Mux2/3
  Mux2/1 -> Slice12/1, Slice11/1, Slice10/1, Slice9/1, Convert2/1
  Logical4/1 -> Logical/2
  Logical5/1 -> Logical4/2
  Logical6/1 -> Logical4/1
  Slice8/1 -> Logical5/3, Logical5/4, Logical6/4
  Slice7/1 -> Logical6/3
  Slice6/1 -> Logical5/2, Logical6/2
  Slice5/1 -> Logical5/1, Logical6/1
  Convert1/1 -> ri_to_c/2
  Scale1/1 -> Mux1/3
  Mux1/1 -> Slice8/1, Slice7/1, Slice6/1, Slice5/1, Convert1/1
  Logical1/1 -> Logical/1
  Logical2/1 -> Logical1/2
  Logical3/1 -> Logical1/1
  Slice4/1 -> Logical2/4, Logical3/4
  Slice3/1 -> Logical2/3, Logical3/3
  Slice2/1 -> Logical2/2, Logical3/2
  Slice1/1 -> Logical2/1, Logical3/1
  Convert/1 -> ri_to_c/1
  Scale/1 -> Mux/3
  Mux/1 -> Slice4/1, Slice3/1, Slice2/1, Slice1/1, Convert/1
  shift/1 -> Delay3/1
  AddSub1/1 -> Scale1/1, Mux1/2
  AddSub/1 -> Scale/1, Mux/2
  Delay/1 -> sync_out/1
  ri_to_c1/1 -> a-bw/1
  ri_to_c/1 -> a+bw/1
  a/1 -> twiddle/1(a)
  b/1 -> twiddle/2(b)
  sync/1 -> twiddle/3(sync)
  twiddle/1(a_re) -> AddSub/1, AddSub2/1
  twiddle/2(a_im) -> AddSub1/1, AddSub3/1
  twiddle/3(bw_re) -> AddSub/2, AddSub2/2
  twiddle/4(bw_im) -> AddSub1/2, AddSub3/2
  twiddle/5(sync_out) -> Delay/1

== system dual500MHzPFB/cfgspec/FFT_Subsystem/fft_wideband_real/fft_biplex_real_4x0/biplex_core/fft_stage_4/delay_b ==
  In1 : Inport  Port=1  LatchInput=off
  delay_slr : casper_library/Delays/delay_slr  DelayLen=2^(FFTSize-FFTStage)
  Out1 : Outport
  wires:
  In1/1 -> delay_slr/1
  delay_slr/1 -> Out1/1

== system dual500MHzPFB/cfgspec/FFT_Subsystem/fft_wideband_real/fft_biplex_real_4x0/biplex_core/fft_stage_4/delay_f ==
  In1 : Inport  Port=1  LatchInput=off
  delay_slr : casper_library/Delays/delay_slr  DelayLen=2^(FFTSize-FFTStage)
  Out1 : Outport
  wires:
  In1/1 -> delay_slr/1
  delay_slr/1 -> Out1/1
